simulink model "Comparison_of_models"  (R2023a)
settings: Solver=ode45  StartTime=0.0  StopTime=1.8  RelTol=1e-30
model workspace (MAT data in the model file):
  N_p0 = 5
  N_v0 = 0
  N_w0 = 0
  t_ion = 0
  t_p = 12
  t_pump = 32
  t_release = 5
  t_retention = 2
settings Model: ParameterArgumentNames=N_p0,N_v0,N_w0,t_ion,t_p,t_pump,t_release,t_retention  Creator=levsi  LastModifiedBy=levsi
settings DataIOCC: ReturnWorkspaceOutputs=off

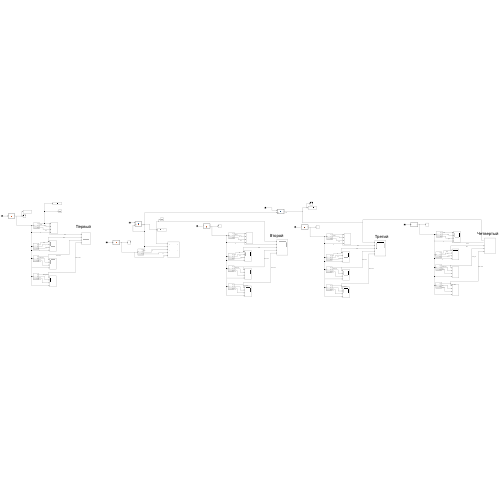
[thumbnail: Simulink's stored preview of the top-level diagram]
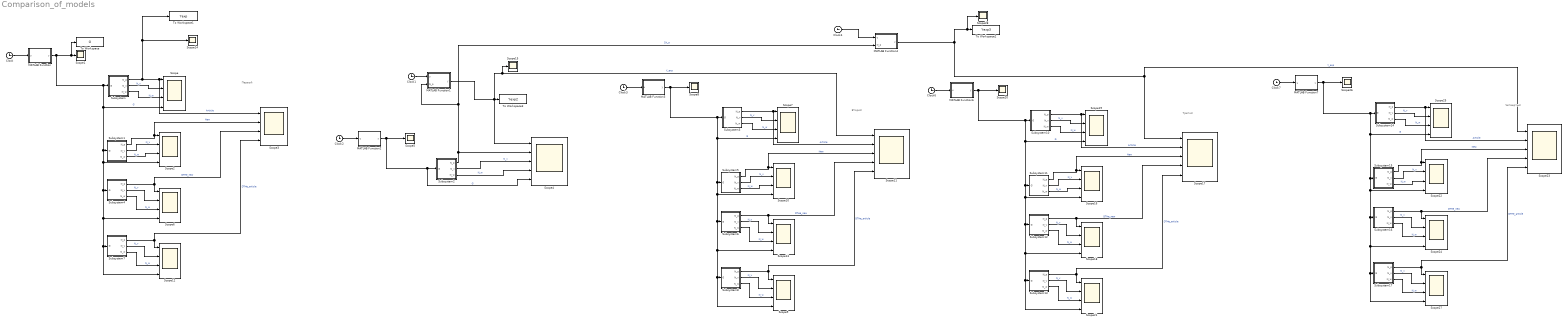
== system Comparison_of_models ==
  note: Четвертый
  note: Третий
  note: Второй
  note: Первый
  Clock{,1..4,6..7} (7 alike) : Clock
  MATLAB Function : MATLAB Function  TreatAsAtomicUnit=on
  MATLAB Function1 : MATLAB Function  TreatAsAtomicUnit=on
  MATLAB Function2 : MATLAB Function  TreatAsAtomicUnit=on
  MATLAB Function3 : MATLAB Function  TreatAsAtomicUnit=on
  MATLAB Function4 : MATLAB Function  TreatAsAtomicUnit=on
  MATLAB Function6 : MATLAB Function  TreatAsAtomicUnit=on
  MATLAB Function7 : MATLAB Function  TreatAsAtomicUnit=on
  Scope{,2..3,6..7,9..10,12..13,16,18..19,21..22,24..25,27} (17 alike) : Scope  NumInputPorts=4
  Scope{1,5,8,14..15,20,26,28} (8 alike) : Scope
  Scope{4,11,17,23} (4 alike) : Scope  NumInputPorts=5
  Subsystem : Subsystem
  Subsystem1 : Subsystem
  Subsystem10 : Subsystem
  Subsystem11 : Subsystem
  Subsystem12 : Subsystem
  Subsystem13 : Subsystem
  Subsystem14 : Subsystem
  Subsystem15 : Subsystem
  Subsystem16 : Subsystem
  Subsystem17 : Subsystem
  Subsystem2 : Subsystem
  Subsystem3 : Subsystem
  Subsystem4 : Subsystem
  Subsystem5 : Subsystem
  Subsystem6 : Subsystem
  Subsystem7 : Subsystem
  Subsystem8 : Subsystem
  To Workspace : ToWorkspace  VariableName=G  SampleTime=0.001
      settings: Save2DSignal=2-D array (concatenate along first dimension)
  To Workspace1 : ToWorkspace  VariableName=Yexp  SampleTime=0.001
      settings: Save2DSignal=2-D array (concatenate along first dimension)
  To Workspace2 : ToWorkspace  VariableName=Yexp3  SampleTime=0.001
      settings: Save2DSignal=2-D array (concatenate along first dimension)
  To Workspace3 : ToWorkspace  VariableName=Yexp2  SampleTime=0.001
      settings: Save2DSignal=2-D array (concatenate along first dimension)
  wires:
  Subsystem/2(N_v) -> Scope/2  "N_v"
  Subsystem/3(N_w) -> Scope/3  "N_w"
  Clock/1 -> MATLAB Function/1(u)
  Subsystem1/3(N_w) -> Scope2/3  "N_w"
  Subsystem1/2(N_v) -> Scope2/2  "N_v"
  Subsystem1/1(N_p) -> Scope3/2, Scope2/1  "New"
  MATLAB Function/1(y) -> Subsystem1/1(G), Subsystem4/1(G), Subsystem7/1(G), Scope12/4, Scope6/4, Scope2/4, Scope/4, Subsystem/1(G), To Workspace/1, Scope1/1  "G"
  Clock1/1 -> MATLAB Function1/1(u)
  Subsystem/1(N_p) -> Scope3/1, Scope/1, Scope14/1, To Workspace1/1  "Article"
  Subsystem4/1(N_p) -> Scope6/1, Scope3/3  "DTHe_new"
  Subsystem2/1(N_p) -> MATLAB Function4/2(N_p), MATLAB Function1/2(N_p), Scope4/2  "1N_p"
  Subsystem2/3(N_w) -> Scope4/4  "N_w"
  MATLAB Function2/1(y) -> Subsystem2/1(G), Scope4/5, Scope5/1  "G"
  Subsystem2/2(N_v) -> Scope4/3  "N_v"
  Clock2/1 -> MATLAB Function2/1(u)
  MATLAB Function1/1(y) -> Scope4/1, Scope15/1, Scope11/1, To Workspace3/1  "Y_exp"
  Subsystem4/2(N_v) -> Scope6/2  "N_v"
  Subsystem4/3(N_w) -> Scope6/3  "N_w"
  Subsystem7/1(N_p) -> Scope3/4, Scope12/1  "DTHe_article"
  Subsystem7/3(N_w) -> Scope12/3  "N_w"
  Subsystem7/2(N_v) -> Scope12/2  "N_v"
  Subsystem8/3(N_w) -> Scope9/3  "N_w"
  Subsystem3/3(N_w) -> Scope7/3  "N_w"
  Subsystem8/1(N_p) -> Scope11/5, Scope9/1  "DTHe_article"
  Subsystem6/3(N_w) -> Scope13/3  "N_w"
  Subsystem6/1(N_p) -> Scope13/1, Scope11/4  "DTHe_new"
  Subsystem3/2(N_v) -> Scope7/2  "N_v"
  Subsystem6/2(N_v) -> Scope13/2  "N_v"
  Subsystem5/1(N_p) -> Scope11/3, Scope10/1  "New"
  Subsystem8/2(N_v) -> Scope9/2  "N_v"
  Clock3/1 -> MATLAB Function3/1(u)
  MATLAB Function3/1(y) -> Subsystem3/1(G), Subsystem5/1(G), Subsystem6/1(G), Subsystem8/1(G), Scope9/4, Scope13/4, Scope10/4, Scope7/4, Scope8/1  "G"
  Subsystem3/1(N_p) -> Scope11/2, Scope7/1  "Article"
  Subsystem5/3(N_w) -> Scope10/3  "N_w"
  Subsystem5/2(N_v) -> Scope10/2  "N_v"
  MATLAB Function4/1(y) -> Scope28/1, To Workspace2/1, Scope23/1, Scope17/1  "Y_exp"
  Clock4/1 -> MATLAB Function4/1(u)
  Clock6/1 -> MATLAB Function6/1(u)
  Subsystem10/1(N_p) -> Scope17/2, Scope19/1  "Article"
  Subsystem11/3(N_w) -> Scope16/3  "N_w"
  Subsystem11/2(N_v) -> Scope16/2  "N_v"
  Subsystem10/2(N_v) -> Scope19/2  "N_v"
  Subsystem12/2(N_v) -> Scope18/2  "N_v"
  Subsystem10/3(N_w) -> Scope19/3  "N_w"
  Subsystem13/2(N_v) -> Scope21/2  "N_v"
  Subsystem11/1(N_p) -> Scope17/3, Scope16/1  "New"
  Subsystem13/3(N_w) -> Scope21/3  "N_w"
  Subsystem13/1(N_p) -> Scope17/5, Scope21/1  "DTHe_article"
  Subsystem12/1(N_p) -> Scope18/1, Scope17/4  "DTHe_new"
  Subsystem12/3(N_w) -> Scope18/3  "N_w"
  MATLAB Function6/1(y) -> Subsystem10/1(G), Subsystem11/1(G), Subsystem12/1(G), Subsystem13/1(G), Scope21/4, Scope18/4, Scope16/4, Scope19/4, Scope20/1  "G"
  MATLAB Function7/1(y) -> Subsystem14/1(G), Subsystem15/1(G), Subsystem16/1(G), Subsystem17/1(G), Scope27/4, Scope24/4, Scope22/4, Scope25/4, Scope26/1  "G"
  Subsystem17/3(N_w) -> Scope27/3  "N_w"
  Subsystem17/1(N_p) -> Scope23/5, Scope27/1  "DTHe_article"
  Subsystem16/1(N_p) -> Scope24/1, Scope23/4  "DTHe_new"
  Subsystem16/3(N_w) -> Scope24/3  "N_w"
  Subsystem14/3(N_w) -> Scope25/3  "N_w"
  Subsystem15/1(N_p) -> Scope23/3, Scope22/1  "New"
  Clock7/1 -> MATLAB Function7/1(u)
  Subsystem17/2(N_v) -> Scope27/2  "N_v"
  Subsystem16/2(N_v) -> Scope24/2  "N_v"
  Subsystem15/2(N_v) -> Scope22/2  "N_v"
  Subsystem14/1(N_p) -> Scope23/2, Scope25/1  "Article"
  Subsystem15/3(N_w) -> Scope22/3  "N_w"
  Subsystem14/2(N_v) -> Scope25/2  "N_v"

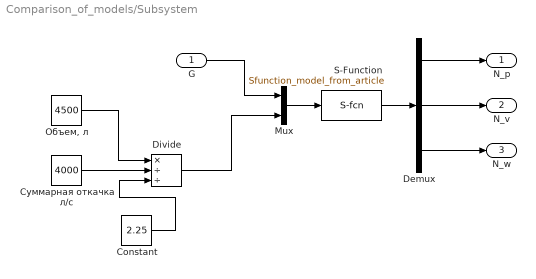
== system Comparison_of_models/Subsystem ==
  G : Inport
  Constant : Constant  Value=2.25
  Demux : Demux  Outputs=3
  Divide : Product  Inputs=*//
  Mux : Mux  Inputs=2
  S-Function : S-Function  FunctionName=Sfunction_model_from_article  Parameters=0.018, 0.01, 0.283, 0.041, 0, 0, 2.5e+18  SFunctionDeploymentMode=off  EnableBusSupport=off
  "Объем, л" : Constant  Value=4500
  Суммарная откачка л/с : Constant  Value=4000
  N_p : Outport
  N_v : Outport  Port=2
  N_w : Outport  Port=3
  wires:
  Demux/1 -> N_p/1
  S-Function/1 -> Demux/1
  Demux/2 -> N_v/1
  Demux/3 -> N_w/1
  Mux/1 -> S-Function/1
  G/1 -> Mux/1
  Divide/1 -> Mux/2
  Constant/1 -> Divide/3
  Суммарная откачка л/с/1 -> Divide/2
  "Объем, л"/1 -> Divide/1

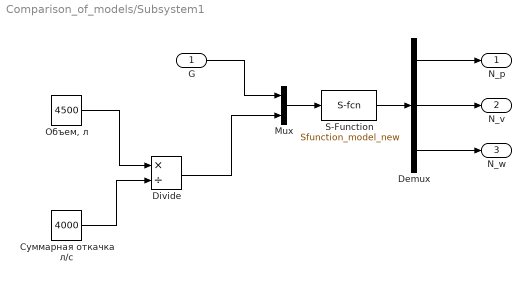
== system Comparison_of_models/Subsystem1 ==
  G : Inport
  Demux : Demux  Outputs=3
  Divide : Product  Inputs=*/
  Mux : Mux  Inputs=2
  S-Function : S-Function  FunctionName=Sfunction_model_new  Parameters=0.0076, 0.0646, 0.2572, 0.0481, 0, 5.1e+18, 2.1e+18  SFunctionDeploymentMode=off  EnableBusSupport=off
  "Объем, л" : Constant  Value=4500
  Суммарная откачка л/с : Constant  Value=4000
  N_p : Outport
  N_v : Outport  Port=2
  N_w : Outport  Port=3
  wires:
  Demux/1 -> N_p/1
  S-Function/1 -> Demux/1
  Demux/2 -> N_v/1
  Demux/3 -> N_w/1
  G/1 -> Mux/1
  Mux/1 -> S-Function/1
  "Объем, л"/1 -> Divide/1
  Divide/1 -> Mux/2
  Суммарная откачка л/с/1 -> Divide/2

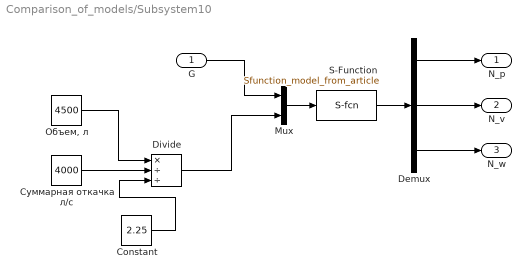
== system Comparison_of_models/Subsystem10 ==
  G : Inport
  Constant : Constant  Value=2.25
  Demux : Demux  Outputs=3
  Divide : Product  Inputs=*//
  Mux : Mux  Inputs=2
  S-Function : S-Function  FunctionName=Sfunction_model_from_article  Parameters=1.5034, 0.0316, 1.9389, 0.1626, 0, 1.455e+20, 0  SFunctionDeploymentMode=off  EnableBusSupport=off
  "Объем, л" : Constant  Value=4500
  Суммарная откачка л/с : Constant  Value=4000
  N_p : Outport
  N_v : Outport  Port=2
  N_w : Outport  Port=3
  wires:
  Demux/1 -> N_p/1
  S-Function/1 -> Demux/1
  Demux/2 -> N_v/1
  Demux/3 -> N_w/1
  G/1 -> Mux/1
  Mux/1 -> S-Function/1
  Constant/1 -> Divide/3
  "Объем, л"/1 -> Divide/1
  Divide/1 -> Mux/2
  Суммарная откачка л/с/1 -> Divide/2

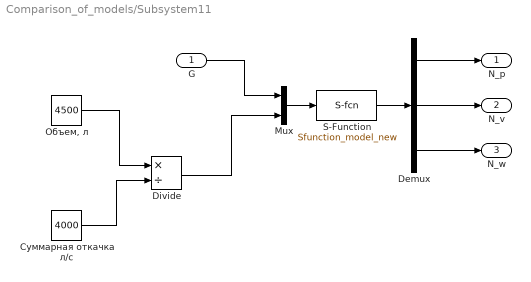
== system Comparison_of_models/Subsystem11 ==
  G : Inport
  Demux : Demux  Outputs=3
  Divide : Product  Inputs=*/
  Mux : Mux  Inputs=2
  S-Function : S-Function  FunctionName=Sfunction_model_new  Parameters=0.0853, 0.0646, 1.709, 0.2245, 0, 1.804e+20, 0  SFunctionDeploymentMode=off  EnableBusSupport=off
  "Объем, л" : Constant  Value=4500
  Суммарная откачка л/с : Constant  Value=4000
  N_p : Outport
  N_v : Outport  Port=2
  N_w : Outport  Port=3
  wires:
  Demux/1 -> N_p/1
  S-Function/1 -> Demux/1
  Demux/2 -> N_v/1
  Demux/3 -> N_w/1
  Суммарная откачка л/с/1 -> Divide/2
  Divide/1 -> Mux/2
  "Объем, л"/1 -> Divide/1
  Mux/1 -> S-Function/1
  G/1 -> Mux/1

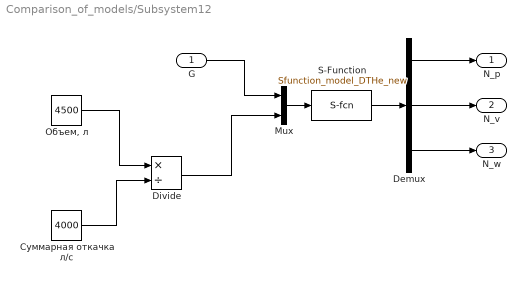
== system Comparison_of_models/Subsystem12 ==
  G : Inport
  Demux : Demux  Outputs=3
  Divide : Product  Inputs=*/
  Mux : Mux  Inputs=2
  S-Function : S-Function  FunctionName=Sfunction_model_DTHe_new  Parameters=0.0068, 5, 0.0884, 0.0251, 0.0289, 0.022, 0.1912, 0.0453, 0.0283, 0, 1, 3.125e+20, 0, 0, 0  SFunctionDeploymentMode=off  EnableBusSupport=off
  "Объем, л" : Constant  Value=4500
  Суммарная откачка л/с : Constant  Value=4000
  N_p : Outport
  N_v : Outport  Port=2
  N_w : Outport  Port=3
  wires:
  Demux/1 -> N_p/1
  S-Function/1 -> Demux/1
  Demux/2 -> N_v/1
  Demux/3 -> N_w/1
  Суммарная откачка л/с/1 -> Divide/2
  Divide/1 -> Mux/2
  "Объем, л"/1 -> Divide/1
  Mux/1 -> S-Function/1
  G/1 -> Mux/1

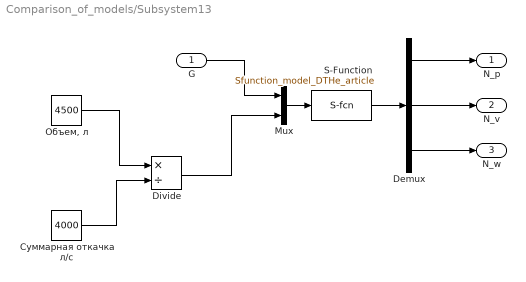
== system Comparison_of_models/Subsystem13 ==
  G : Inport
  Demux : Demux  Outputs=3
  Divide : Product  Inputs=*/
  Mux : Mux  Inputs=2
  S-Function : S-Function  FunctionName=Sfunction_model_DTHe_article  Parameters=0.0035, 5, 0.1129, 0.0095, 0.0069, 0.0166, 0.238, 0.0075, 0.0538, 0, 1, 3.125e+20, 0, 0, 0  SFunctionDeploymentMode=off  EnableBusSupport=off
  "Объем, л" : Constant  Value=4500
  Суммарная откачка л/с : Constant  Value=4000
  N_p : Outport
  N_v : Outport  Port=2
  N_w : Outport  Port=3
  wires:
  Demux/1 -> N_p/1
  S-Function/1 -> Demux/1
  Demux/2 -> N_v/1
  Demux/3 -> N_w/1
  Суммарная откачка л/с/1 -> Divide/2
  Divide/1 -> Mux/2
  "Объем, л"/1 -> Divide/1
  Mux/1 -> S-Function/1
  G/1 -> Mux/1

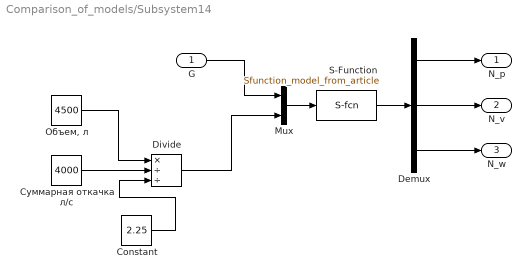
== system Comparison_of_models/Subsystem14 ==
  G : Inport
  Constant : Constant  Value=2.25
  Demux : Demux  Outputs=3
  Divide : Product  Inputs=*//
  Mux : Mux  Inputs=2
  S-Function : S-Function  FunctionName=Sfunction_model_from_article  Parameters=1.5034, 0.0316, 1.9389, 0.1626, 0, 1.455e+20, 0  SFunctionDeploymentMode=off  EnableBusSupport=off
  "Объем, л" : Constant  Value=4500
  Суммарная откачка л/с : Constant  Value=4000
  N_p : Outport
  N_v : Outport  Port=2
  N_w : Outport  Port=3
  wires:
  Demux/1 -> N_p/1
  S-Function/1 -> Demux/1
  Demux/2 -> N_v/1
  Demux/3 -> N_w/1
  G/1 -> Mux/1
  Mux/1 -> S-Function/1
  Constant/1 -> Divide/3
  "Объем, л"/1 -> Divide/1
  Divide/1 -> Mux/2
  Суммарная откачка л/с/1 -> Divide/2

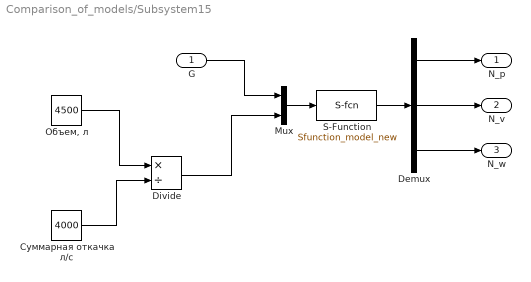
== system Comparison_of_models/Subsystem15 ==
  G : Inport
  Demux : Demux  Outputs=3
  Divide : Product  Inputs=*/
  Mux : Mux  Inputs=2
  S-Function : S-Function  FunctionName=Sfunction_model_new  Parameters=0.0853, 0.0646, 1.709, 0.2245, 0, 1.804e+20, 0  SFunctionDeploymentMode=off  EnableBusSupport=off
  "Объем, л" : Constant  Value=4500
  Суммарная откачка л/с : Constant  Value=4000
  N_p : Outport
  N_v : Outport  Port=2
  N_w : Outport  Port=3
  wires:
  Demux/1 -> N_p/1
  S-Function/1 -> Demux/1
  Demux/2 -> N_v/1
  Demux/3 -> N_w/1
  Суммарная откачка л/с/1 -> Divide/2
  Divide/1 -> Mux/2
  "Объем, л"/1 -> Divide/1
  Mux/1 -> S-Function/1
  G/1 -> Mux/1

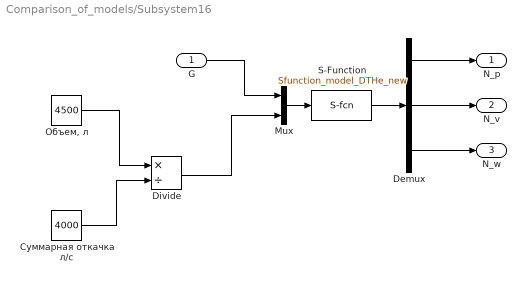
== system Comparison_of_models/Subsystem16 ==
  G : Inport
  Demux : Demux  Outputs=3
  Divide : Product  Inputs=*/
  Mux : Mux  Inputs=2
  S-Function : S-Function  FunctionName=Sfunction_model_DTHe_new  Parameters=0.0073, 5.101e+9, 0.0934, 0.0257, 0.0287 0.022, 0.1926, 0.045, 0.0283, 0, 1, 3.125e+20, 0, 0, 0  SFunctionDeploymentMode=off  EnableBusSupport=off
  "Объем, л" : Constant  Value=4500
  Суммарная откачка л/с : Constant  Value=4000
  N_p : Outport
  N_v : Outport  Port=2
  N_w : Outport  Port=3
  wires:
  Demux/1 -> N_p/1
  S-Function/1 -> Demux/1
  Demux/2 -> N_v/1
  Demux/3 -> N_w/1
  Суммарная откачка л/с/1 -> Divide/2
  Divide/1 -> Mux/2
  "Объем, л"/1 -> Divide/1
  Mux/1 -> S-Function/1
  G/1 -> Mux/1

== system Comparison_of_models/Subsystem17 ==
  G : Inport
  Demux : Demux  Outputs=3
  Divide : Product  Inputs=*/
  Mux : Mux  Inputs=2
  S-Function : S-Function  FunctionName=Sfunction_model_DTHe_article  Parameters=0.0037, 5.366, 0.1144, 0.01, 0.0067, 0.0165, 0.24, 0.0067, 0.0539, 0, 1, 3.125e+20, 0, 0, 0  SFunctionDeploymentMode=off  EnableBusSupport=off
  "Объем, л" : Constant  Value=4500
  Суммарная откачка л/с : Constant  Value=4000
  N_p : Outport
  N_v : Outport  Port=2
  N_w : Outport  Port=3
  wires:
  Demux/1 -> N_p/1
  S-Function/1 -> Demux/1
  Demux/2 -> N_v/1
  Demux/3 -> N_w/1
  Суммарная откачка л/с/1 -> Divide/2
  Divide/1 -> Mux/2
  "Объем, л"/1 -> Divide/1
  Mux/1 -> S-Function/1
  G/1 -> Mux/1

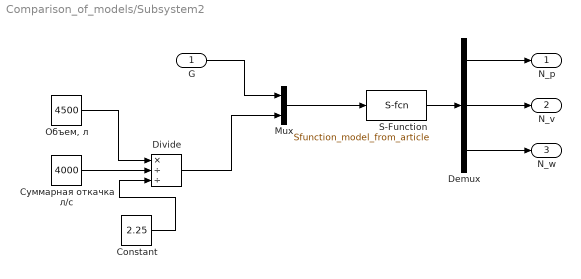
== system Comparison_of_models/Subsystem2 ==
  G : Inport
  Constant : Constant  Value=2.25
  Demux : Demux  Outputs=3
  Divide : Product  Inputs=*//
  Mux : Mux  Inputs=2
  S-Function : S-Function  FunctionName=Sfunction_model_from_article  Parameters=0.018, 0.01, 0.283, 0.041, 0, 0, 2.5e+18  SFunctionDeploymentMode=off  EnableBusSupport=off
  "Объем, л" : Constant  Value=4500
  Суммарная откачка л/с : Constant  Value=4000
  N_p : Outport
  N_v : Outport  Port=2
  N_w : Outport  Port=3
  wires:
  Demux/1 -> N_p/1
  S-Function/1 -> Demux/1
  Demux/2 -> N_v/1
  Demux/3 -> N_w/1
  G/1 -> Mux/1
  Mux/1 -> S-Function/1
  Constant/1 -> Divide/3
  "Объем, л"/1 -> Divide/1
  Divide/1 -> Mux/2
  Суммарная откачка л/с/1 -> Divide/2

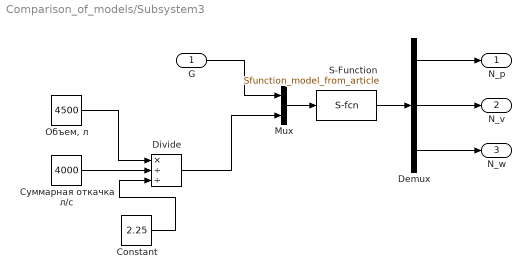
== system Comparison_of_models/Subsystem3 ==
  G : Inport
  Constant : Constant  Value=2.25
  Demux : Demux  Outputs=3
  Divide : Product  Inputs=*//
  Mux : Mux  Inputs=2
  S-Function : S-Function  FunctionName=Sfunction_model_from_article  Parameters=5, 0.0322, 1.8578, 0.1827, 0, 1.601e+20, 0  SFunctionDeploymentMode=off  EnableBusSupport=off
  "Объем, л" : Constant  Value=4500
  Суммарная откачка л/с : Constant  Value=4000
  N_p : Outport
  N_v : Outport  Port=2
  N_w : Outport  Port=3
  wires:
  Demux/1 -> N_p/1
  S-Function/1 -> Demux/1
  Demux/2 -> N_v/1
  Demux/3 -> N_w/1
  G/1 -> Mux/1
  Mux/1 -> S-Function/1
  Constant/1 -> Divide/3
  "Объем, л"/1 -> Divide/1
  Divide/1 -> Mux/2
  Суммарная откачка л/с/1 -> Divide/2

== system Comparison_of_models/Subsystem4 ==
  G : Inport
  Demux : Demux  Outputs=3
  Divide : Product  Inputs=*/
  Mux : Mux  Inputs=2
  S-Function : S-Function  FunctionName=Sfunction_model_DTHe_new  Parameters=0.0051, 0.0389, 0.2732, 0.0122, 0.0429, 0.03, 0.1545, 0.0628, 0.0323, 0, 1, 1e+18, 0, 0, 0  SFunctionDeploymentMode=off  EnableBusSupport=off
  "Объем, л" : Constant  Value=4500
  Суммарная откачка л/с : Constant  Value=4000
  N_p : Outport
  N_v : Outport  Port=2
  N_w : Outport  Port=3
  wires:
  Demux/1 -> N_p/1
  S-Function/1 -> Demux/1
  Demux/2 -> N_v/1
  Demux/3 -> N_w/1
  Суммарная откачка л/с/1 -> Divide/2
  Divide/1 -> Mux/2
  "Объем, л"/1 -> Divide/1
  Mux/1 -> S-Function/1
  G/1 -> Mux/1

== system Comparison_of_models/Subsystem5 ==
  G : Inport
  Demux : Demux  Outputs=3
  Divide : Product  Inputs=*/
  Mux : Mux  Inputs=2
  S-Function : S-Function  FunctionName=Sfunction_model_new  Parameters=0.0995, 0.0622, 1.4499, 0.2699, 0, 2.163e+20, 0  SFunctionDeploymentMode=off  EnableBusSupport=off
  "Объем, л" : Constant  Value=4500
  Суммарная откачка л/с : Constant  Value=4000
  N_p : Outport
  N_v : Outport  Port=2
  N_w : Outport  Port=3
  wires:
  Demux/1 -> N_p/1
  S-Function/1 -> Demux/1
  Demux/2 -> N_v/1
  Demux/3 -> N_w/1
  Суммарная откачка л/с/1 -> Divide/2
  Divide/1 -> Mux/2
  "Объем, л"/1 -> Divide/1
  Mux/1 -> S-Function/1
  G/1 -> Mux/1

== system Comparison_of_models/Subsystem6 ==
  G : Inport
  Demux : Demux  Outputs=3
  Divide : Product  Inputs=*/
  Mux : Mux  Inputs=2
  S-Function : S-Function  FunctionName=Sfunction_model_DTHe_new  Parameters=0.0062, 5, 0.0806, 0.0259, 0.03, 0.0223, 0.1899, 0.0457, 0.0271, 0, 1, 3.087e+20, 0, 0, 0  SFunctionDeploymentMode=off  EnableBusSupport=off
  "Объем, л" : Constant  Value=4500
  Суммарная откачка л/с : Constant  Value=4000
  N_p : Outport
  N_v : Outport  Port=2
  N_w : Outport  Port=3
  wires:
  Demux/1 -> N_p/1
  S-Function/1 -> Demux/1
  Demux/2 -> N_v/1
  Demux/3 -> N_w/1
  Суммарная откачка л/с/1 -> Divide/2
  Divide/1 -> Mux/2
  "Объем, л"/1 -> Divide/1
  Mux/1 -> S-Function/1
  G/1 -> Mux/1

== system Comparison_of_models/Subsystem7 ==
  G : Inport
  Demux : Demux  Outputs=3
  Divide : Product  Inputs=*/
  Mux : Mux  Inputs=2
  S-Function : S-Function  FunctionName=Sfunction_model_DTHe_article  Parameters=0.0026, 0.1006, 0.7133, 0.0085, 0.0251, 0.0294, 0.1597, 0.0547, 0.0248, 0, 1, 1, 0, 0, 0  SFunctionDeploymentMode=off  EnableBusSupport=off
  "Объем, л" : Constant  Value=4500
  Суммарная откачка л/с : Constant  Value=4000
  N_p : Outport
  N_v : Outport  Port=2
  N_w : Outport  Port=3
  wires:
  Demux/1 -> N_p/1
  S-Function/1 -> Demux/1
  Demux/2 -> N_v/1
  Demux/3 -> N_w/1
  Суммарная откачка л/с/1 -> Divide/2
  Divide/1 -> Mux/2
  "Объем, л"/1 -> Divide/1
  Mux/1 -> S-Function/1
  G/1 -> Mux/1

== system Comparison_of_models/Subsystem8 ==
  G : Inport
  Demux : Demux  Outputs=3
  Divide : Product  Inputs=*/
  Mux : Mux  Inputs=2
  S-Function : S-Function  FunctionName=Sfunction_model_DTHe_article  Parameters=0.0041, 5, 0.104, 0.0122, 0.0078, 0.0171, 0.2331, 0.0072, 0.0532, 0, 1, 3.087e+20, 0, 0, 0  SFunctionDeploymentMode=off  EnableBusSupport=off
  "Объем, л" : Constant  Value=4500
  Суммарная откачка л/с : Constant  Value=4000
  N_p : Outport
  N_v : Outport  Port=2
  N_w : Outport  Port=3
  wires:
  Demux/1 -> N_p/1
  S-Function/1 -> Demux/1
  Demux/2 -> N_v/1
  Demux/3 -> N_w/1
  Суммарная откачка л/с/1 -> Divide/2
  Divide/1 -> Mux/2
  "Объем, л"/1 -> Divide/1
  Mux/1 -> S-Function/1
  G/1 -> Mux/1

== matlab function Comparison_of_models/MATLAB Function ==
  data: u input; y output
function y = fcn(u)

if (0<=u) && (u<0.2)
    y = (-4e+22)*u^2 + (5e+21)*u + (1.25e+21);
elseif (0.2<=u) && (u<0.5)
    y = 7.62*10^20;
elseif (0.5<=u && u<0.7) || (0.77<=u && u<0.8) || (0.92<=u && u<1.07) || (1.12<=u && u<1.17) || (1.23<=u && u<1.37) || (1.54<=u && u<1.59) 
    y = 2.162*10^20;
elseif (0.7<=u && u<0.77) || (0.8<=u && u<0.92) || (1.07<=u && u<1.12) || (1.17<=u && u<1.23) || (1.37<=u && u<1.54)
    y = 1.27*10^21;
elseif (1.59<=u && u<1.61)
    y = 7.027*10^20;
else
    y = 0;
end

end

== matlab function Comparison_of_models/MATLAB Function2 ==
  data: u input; y output
function y = fcn(u)

if (0<=u) && (u<0.2)
    y = (-4e+22)*u^2 + (5e+21)*u + (1.25e+21);
elseif (0.2<=u) && (u<0.5)
    y = 7.62*10^20;
elseif (0.5<=u && u<0.7) || (0.77<=u && u<0.8) || (0.92<=u && u<1.07) || (1.12<=u && u<1.17) || (1.23<=u && u<1.37) || (1.54<=u && u<1.59) 
    y = 2.162*10^20;
elseif (0.7<=u && u<0.77) || (0.8<=u && u<0.92) || (1.07<=u && u<1.12) || (1.17<=u && u<1.23) || (1.37<=u && u<1.54)
    y = 1.27*10^21;
elseif (1.59<=u && u<1.61)
    y = 7.027*10^20;
else
    y = 0;
end

end

== matlab function Comparison_of_models/MATLAB Function3 ==
  data: u input; y output
function y = fcn(u)

if (0<=u) && (u<0.2)
    y = (-4e+22)*u^2 + (5e+21)*u + (1.25e+21);
elseif (0.2<=u) && (u<0.5)
    y = 7.62*10^20;
elseif (0.5<=u && u<0.7) || (0.77<=u && u<0.8) || (0.92<=u && u<1.07) || (1.12<=u && u<1.17) || (1.23<=u && u<1.37) || (1.54<=u && u<1.59) 
    y = 2.162*10^20;
elseif (0.7<=u && u<0.77) || (0.8<=u && u<0.92) || (1.07<=u && u<1.12) || (1.17<=u && u<1.23) || (1.37<=u && u<1.54)
    y = 1.27*10^21;
elseif (1.59<=u && u<1.61)
    y = 7.027*10^20;
else
    y = 0;
end

end

== matlab function Comparison_of_models/MATLAB Function4 ==
  data: u input; y output; N_p input
function y  = fcn(u, N_p)

if (0<=u) && (u<0.53)
    y = 390.98*u^3 - 429.25*u^2 + 117.8*u - 0.3215;
    y = y*(5*10^18);
    y = N_p + y;
elseif (0.53<=u) && (u<1.62)
    y = N_p;
elseif u>=1.62
    y= -28948929495286300000000*u^3 + 145674489317660000000000*u^2 - 244339807909725000000000*u + 136666492567801000000000;
else 
    y = 0;
end

if y<0
    y = 0;
end

end

== matlab function Comparison_of_models/MATLAB Function6 ==
  data: u input; y output
function y = fcn(u)

if (0<=u) && (u<0.2)
    y = (-4e+22)*u^2 + (5e+21)*u + (1.25e+21);
elseif (0.2<=u) && (u<0.5)
    y = 7.62*10^20;
elseif (0.5<=u && u<0.7) || (0.77<=u && u<0.8) || (0.92<=u && u<1.07) || (1.12<=u && u<1.17) || (1.23<=u && u<1.37) || (1.54<=u && u<1.59) 
    y = 2.162*10^20;
elseif (0.7<=u && u<0.77) || (0.8<=u && u<0.92) || (1.07<=u && u<1.12) || (1.17<=u && u<1.23) || (1.37<=u && u<1.54)
    y = 1.27*10^21;
elseif (1.59<=u && u<1.61)
    y = 7.027*10^20;
else
    y = 0;
end

end

== matlab function Comparison_of_models/MATLAB Function7 ==
  data: u input; y output
function y = fcn(u)

if (0<=u) && (u<0.2)
    y = (-4e+22)*u^2 + (5e+21)*u + (1.25e+21);
elseif (0.2<=u) && (u<0.5)
    y = 7.62*10^20;
elseif (0.5<=u && u<0.7) || (0.77<=u && u<0.8) || (0.92<=u && u<1.07) || (1.12<=u && u<1.17) || (1.23<=u && u<1.37) || (1.54<=u && u<1.59) 
    y = 2.162*10^20;
elseif (0.7<=u && u<0.77) || (0.8<=u && u<0.92) || (1.07<=u && u<1.12) || (1.17<=u && u<1.23) || (1.37<=u && u<1.54)
    y = 1.27*10^21;
elseif (1.59<=u && u<1.61)
    y = 7.027*10^20;
else
    y = 0;
end

end

== matlab function Comparison_of_models/MATLAB Function1 ==
  data: u input; y output; N_p input
function y  = fcn(u, N_p)

if (0<=u) && (u<0.53)
    y = 390.98*u^3 - 429.25*u^2 + 117.8*u - 0.3215;
    y = y*(5*10^18);
    y = N_p + y;
elseif (0.53<=u) && (u<1.61)
    y = N_p;
elseif u>=1.61
    y= (-4.173822371660780e+22)*u^3 + (2.076070085717630e+23)*u^2 - (3.439743933468400e+23)*u + 1.899107156750840e+23;
else 
    y = 0;
end

if y<0
    y = 0;
end

end
